simulink model "Position_Controller_V3"  (Simulink 8.9)
settings: Solver=VariableStepAuto  StartTime=0.0  StopTime=1  MaxStep=0.01  RelTol=1e-4  EnableMultiTasking=on
settings Model: Creator=MONSTER  LastModifiedBy=MONSTER
settings SolverCC: ZeroCrossAlgorithm=Adaptive
settings DataIOCC: SaveFormat=Dataset  SignalLoggingSaveFormat=Dataset  SaveOutput=off  SaveTime=off
settings OptimizationCC: ExpressionDepthLimit=2147483647  LifeSpan=1
settings DebuggingCC: AllowSymbolicDim=off
settings HardwareCC: ProdBitPerPointer=64  ProdBitPerSizeT=64  ProdBitPerPtrDiffT=64  ProdLargestAtomicFloat=Float  ProdIntDivRoundTo=Zero  ProdEndianess=LittleEndian  ProdWordSize=64  ProdHWDeviceType=Intel->x86-64 (Windows64)
settings ModelReferenceCC: PropagateSignalLabelsOutOfModel=on
settings ConfigComp: CovMetricSettings=dwe  CovHtmlReporting=off  CovSaveCumulativeToWorkspaceVar=off  CovSaveSingleToWorkspaceVar=off  CovExternalEMLEnable=on

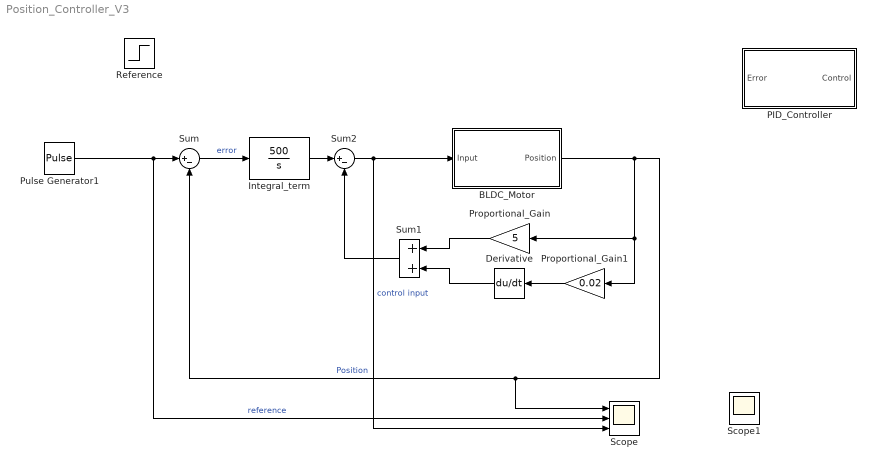
== system Position_Controller_V3 ==
  BLDC_Motor : Subsystem
  Derivative : Derivative
  "Integral_term " : TransferFcn  Numerator=500  Denominator=[1 0]
  PID_Controller : Subsystem
  Proportional_Gain : Gain  Gain=5
  Proportional_Gain1 : Gain  Gain=0.02
  Pulse Generator1 : DiscretePulseGenerator  PulseType=Time based  Period=0.2  PulseWidth=60
  Reference : Step  Time=0.1  After=5  SampleTime=0
  Scope : Scope  NumInputPorts=3
  Scope1 : Scope
  Sum : Sum  Inputs=|+-
  Sum1 : Sum
  Sum2 : Sum  Inputs=|+-
  wires:
  Pulse Generator1/1 -> Scope/2, Sum/1  "reference"
  BLDC_Motor/1(Position) -> Proportional_Gain/1, Proportional_Gain1/1, Sum/2, Scope/1  "Position"
  Sum/1 -> "Integral_term "/1  "error"
  Sum2/1 -> Scope/3, BLDC_Motor/1(Input)  "control input"
  "Integral_term "/1 -> Sum2/1
  Proportional_Gain1/1 -> Derivative/1
  Derivative/1 -> Sum1/2
  Proportional_Gain/1 -> Sum1/1
  Sum1/1 -> Sum2/2

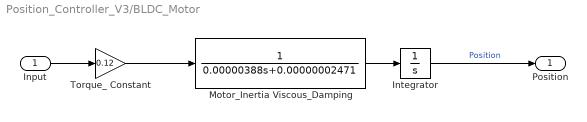
== system Position_Controller_V3/BLDC_Motor ==
  Input : Inport
  Integrator : Integrator
  Motor_Inertia Viscous_Damping : TransferFcn  Denominator=[0.00000388 0.00000002471]
  Torque_ Constant : Gain  Gain=0.12
  Position : Outport
  wires:
  Input/1 -> Torque_ Constant/1
  Integrator/1 -> Position/1  "Position"
  Motor_Inertia Viscous_Damping/1 -> Integrator/1
  Torque_ Constant/1 -> Motor_Inertia Viscous_Damping/1

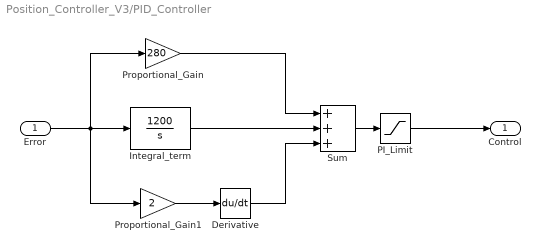
== system Position_Controller_V3/PID_Controller ==
  Error : Inport
  Derivative : Derivative
  "Integral_term " : TransferFcn  Numerator=1200  Denominator=[1 0]
  PI_Limit : Saturate  UpperLimit=1  LowerLimit=-1
  Proportional_Gain : Gain  Gain=280
  Proportional_Gain1 : Gain  Gain=2
  Sum : Sum  Inputs=+++
  Control : Outport
  wires:
  PI_Limit/1 -> Control/1
  Proportional_Gain/1 -> Sum/1
  "Integral_term "/1 -> Sum/2
  Derivative/1 -> Sum/3
  Sum/1 -> PI_Limit/1
  Proportional_Gain1/1 -> Derivative/1
  Error/1 -> Proportional_Gain/1, "Integral_term "/1, Proportional_Gain1/1
